simulink model "simulink_test"  (R2022b)
settings: Solver=VariableStepAuto  StartTime=0.0  StopTime=200000  RelTol=1e-3
undefined symbols (not defined in the file): m, n
settings Model: Creator=pedro  LastModifiedBy=pedro

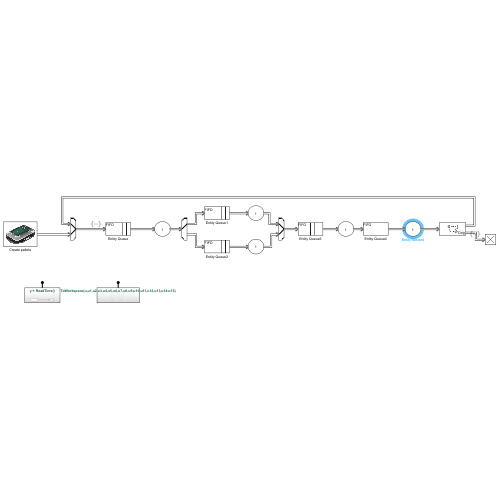
[thumbnail: Simulink's stored preview of the top-level diagram]
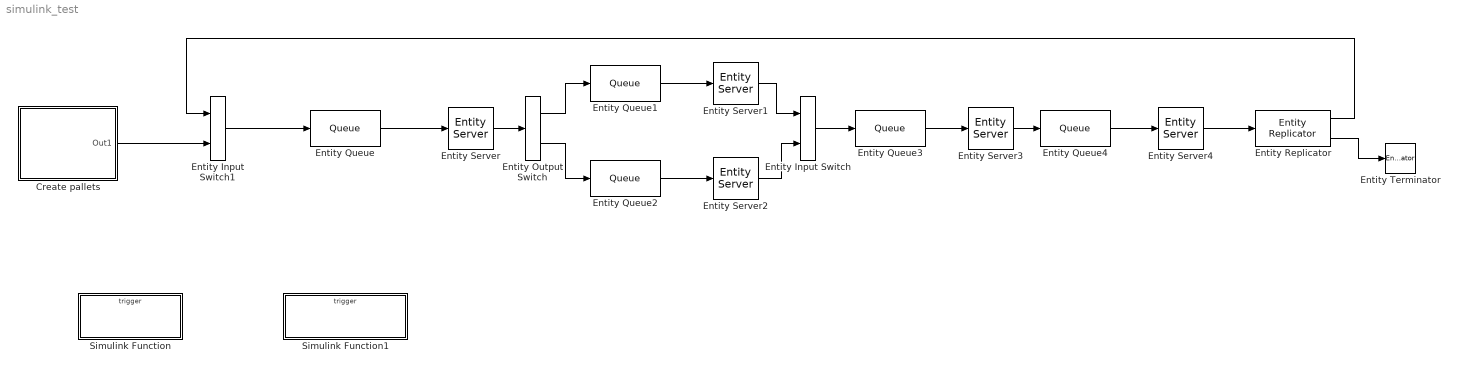
== system simulink_test ==
  Create pallets : Subsystem
      mask Display: image('$imagefile'); % Use "Edit Image" on toolstrip to change.
  Entity Input Switch : EntityInputSwitch  InputPortMessageModes=m,m  OutputPortMessageModes=m
  Entity Input Switch1 : EntityInputSwitch  InputPortMessageModes=m,m  OutputPortMessageModes=m
  Entity Output Switch : EntityOutputSwitch  InputPortMessageModes=m  OutputPortMessageModes=m,m  SwitchAttributeName=Attribute1
  Entity Queue : Queue  InputPortMessageModes=m  OutputPortMessageModes=m  Capacity=100  EntryAction=entity.Time_In_System = ReadTime();
  Entity Queue1 : Queue  InputPortMessageModes=m  OutputPortMessageModes=m  Capacity=3
  Entity Queue2 : Queue  InputPortMessageModes=m  OutputPortMessageModes=m  Capacity=7
  Entity Queue3 : Queue  InputPortMessageModes=m  OutputPortMessageModes=m  Capacity=20
  Entity Queue4 : Queue  InputPortMessageModes=m  OutputPortMessageModes=m  Capacity=10
  Entity Replicator : EntityReplicator  InputPortMessageModes=m  OutputPortMessageModes=m,m
  Entity Server : EntityServer  InputPortMessageModes=m  OutputPortMessageModes=m  Capacity=1  ServiceTimeValue=5000
  Entity Server1 : EntityServer  InputPortMessageModes=m  OutputPortMessageModes=m  Capacity=1  ServiceTimeValue=15000
  Entity Server2 : EntityServer  InputPortMessageModes=m  OutputPortMessageModes=m  Capacity=1  ServiceTimeValue=15000
  Entity Server3 : EntityServer  InputPortMessageModes=m  OutputPortMessageModes=m  Capacity=1  ServiceTimeValue=5000
  Entity Server4 : EntityServer  InputPortMessageModes=m  OutputPortMessageModes=m  Capacity=1  ServiceTimeValue=10000
  Entity Terminator : EntityTerminator  InputPortMessageModes=m  EntryAction=|
      | entity.Time_Out_System = ReadTime();
      | ToWorkspace(entity.Time_In_System,entity.Time_In_Cover, entity.Time_In_Drill, entity.Time_In_Robot, entity.Time_In_Camera, entity.Time_In_Back, entity.Time_In_Press, entity.Time_In_Manual, entity.Time_Out_System, entity.Time_Out_Cover, entity.Time_Out_Drill, entity.Time_Out_Robot, entity.Time_Out_Camera, entity.Time_Out_Back, entity.Time_Out_Press, entity.Time_Out_Manual)
  Simulink Function : Subsystem  TreatAsAtomicUnit=on
  Simulink Function1 : Subsystem  TreatAsAtomicUnit=on
  wires:
  Entity Queue/1 -> Entity Server/1
  Entity Server/1 -> Entity Output Switch/1
  Entity Output Switch/1 -> Entity Queue1/1
  Entity Output Switch/2 -> Entity Queue2/1
  Entity Queue1/1 -> Entity Server1/1
  Entity Queue2/1 -> Entity Server2/1
  Entity Server1/1 -> Entity Input Switch/1
  Entity Server2/1 -> Entity Input Switch/2
  Entity Input Switch/1 -> Entity Queue3/1
  Entity Queue3/1 -> Entity Server3/1
  Entity Server3/1 -> Entity Queue4/1
  Entity Queue4/1 -> Entity Server4/1
  Create pallets/1(Out1) -> Entity Input Switch1/2
  Entity Input Switch1/1 -> Entity Queue/1
  Entity Server4/1 -> Entity Replicator/1
  Entity Replicator/2 -> Entity Terminator/1
  Entity Replicator/1 -> Entity Input Switch1/1

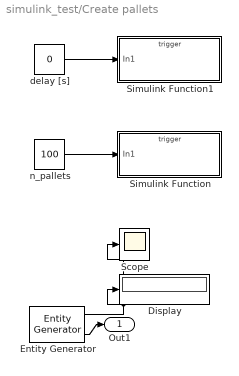
== system simulink_test/Create pallets ==
  Display : Display
  Entity Generator : EntityGenerator  OutputPortMessageModes=n,m  TimeSource=MATLAB action  IntergenerationTimeAction=|  GenerateEntityAtSimulationStart=off  GenerateAction=|  AttributeName=ID|Time_In_Cover|Time_Out_Cover|Time_In_Drill|Time_Out_Drill|Time_In_Robot|Time_Out_Robot|Time_In_Camera|Time_Out_Camera|Time_In_Back|Time_Out_Back|Time_In_Press|Time_Out_Press|Time_In_Manual|Time_Out_Manual|Time_Exit_Cover|Time_In_System|Time_Out_System|Queue1_capacity|Queue2_capacity|Queue3_capacity|Queue4_capacity|Queue5_capacity|Queue6_capacity|Queue1_time|Queue2_time|Queue3_time|Queue4_time|Queue5_time|Queue6_time|data30  AttributeInitialValue=1|0|0|0|0|0|0|0|0|0|0|0|0|0|0|0|0|0|1|1|1|1|1|1|1|1|1|1|1|1|1  NumberEntitiesDeparted=on  EntityType=Structured  EntityTypeName=Entity
      IntergenerationTimeAction=|
      | persistent count
      | if isempty(count)
      |     count = 1;
      | else
      |     count = count + 1;
      | end
      | dt = 0;
      | if count == 1
      |     dt = delay();
      | elseif count > n_pallets()
      |     dt = inf;
      | end
      GenerateAction=|
      | persistent count
      | if isempty(count)
      |     count = 1;
      | else
      |     count = count + 1;
      | end
      | entity.ID = count;
      settings: OutputPortMap=o0,o3
  Scope : Scope
  Simulink Function : Subsystem  TreatAsAtomicUnit=on
  Simulink Function1 : Subsystem  TreatAsAtomicUnit=on
  delay [s] : Constant  Value=0
  n_pallets : Constant  Value=100
  Out1 : Outport
  wires:
  Entity Generator/2 -> Out1/1
  Entity Generator/1 -> Display/1, Scope/1
  n_pallets/1 -> Simulink Function/1(In1)
  delay [s]/1 -> Simulink Function1/1(In1)

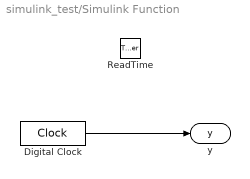
== system simulink_test/Simulink Function ==
  ReadTime : TriggerPort  TriggerType=function-call  IsSimulinkFunction=on  FunctionName=ReadTime  FunctionVisibility=scoped  VariantControl=(inherit)
  Digital Clock : DigitalClock  SampleTime=-1
  y : ArgOut  DisableCoverage=on  ArgumentName=y
  wires:
  Digital Clock/1 -> y/1

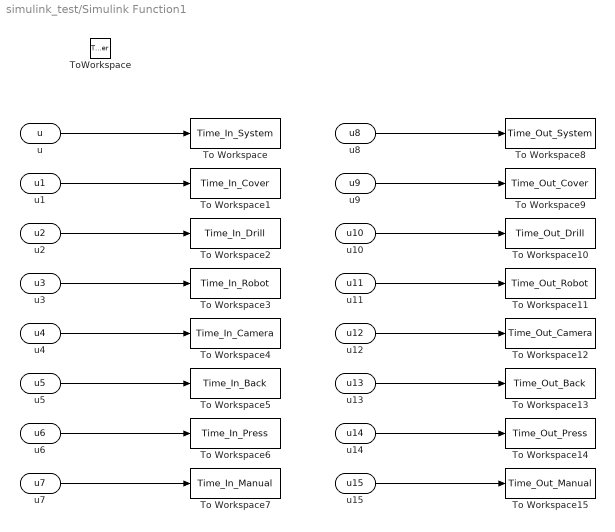
== system simulink_test/Simulink Function1 ==
  ToWorkspace : TriggerPort  TriggerType=function-call  IsSimulinkFunction=on  FunctionName=ToWorkspace  FunctionVisibility=scoped  VariantControl=(inherit)
  To Workspace : ToWorkspace  VariableName=Time_In_System  SampleTime=-1
      settings: Save2DSignal=2-D array (concatenate along first dimension)
  To Workspace1 : ToWorkspace  VariableName=Time_In_Cover  SampleTime=-1
      settings: Save2DSignal=2-D array (concatenate along first dimension)
  To Workspace10 : ToWorkspace  VariableName=Time_Out_Drill  SampleTime=-1
      settings: Save2DSignal=2-D array (concatenate along first dimension)
  To Workspace11 : ToWorkspace  VariableName=Time_Out_Robot  SampleTime=-1
      settings: Save2DSignal=2-D array (concatenate along first dimension)
  To Workspace12 : ToWorkspace  VariableName=Time_Out_Camera  SampleTime=-1
      settings: Save2DSignal=2-D array (concatenate along first dimension)
  To Workspace13 : ToWorkspace  VariableName=Time_Out_Back  SampleTime=-1
      settings: Save2DSignal=2-D array (concatenate along first dimension)
  To Workspace14 : ToWorkspace  VariableName=Time_Out_Press  SampleTime=-1
      settings: Save2DSignal=2-D array (concatenate along first dimension)
  To Workspace15 : ToWorkspace  VariableName=Time_Out_Manual  SampleTime=-1
      settings: Save2DSignal=2-D array (concatenate along first dimension)
  To Workspace2 : ToWorkspace  VariableName=Time_In_Drill  SampleTime=-1
      settings: Save2DSignal=2-D array (concatenate along first dimension)
  To Workspace3 : ToWorkspace  VariableName=Time_In_Robot  SampleTime=-1
      settings: Save2DSignal=2-D array (concatenate along first dimension)
  To Workspace4 : ToWorkspace  VariableName=Time_In_Camera  SampleTime=-1
      settings: Save2DSignal=2-D array (concatenate along first dimension)
  To Workspace5 : ToWorkspace  VariableName=Time_In_Back  SampleTime=-1
      settings: Save2DSignal=2-D array (concatenate along first dimension)
  To Workspace6 : ToWorkspace  VariableName=Time_In_Press  SampleTime=-1
      settings: Save2DSignal=2-D array (concatenate along first dimension)
  To Workspace7 : ToWorkspace  VariableName=Time_In_Manual  SampleTime=-1
      settings: Save2DSignal=2-D array (concatenate along first dimension)
  To Workspace8 : ToWorkspace  VariableName=Time_Out_System  SampleTime=-1
      settings: Save2DSignal=2-D array (concatenate along first dimension)
  To Workspace9 : ToWorkspace  VariableName=Time_Out_Cover  SampleTime=-1
      settings: Save2DSignal=2-D array (concatenate along first dimension)
  u : ArgIn  DisableCoverage=on  ArgumentName=u
  u1 : ArgIn  DisableCoverage=on  Port=2  ArgumentName=u1
  u2 : ArgIn  DisableCoverage=on  Port=3  ArgumentName=u2
  u3 : ArgIn  DisableCoverage=on  Port=4  ArgumentName=u3
  u4 : ArgIn  DisableCoverage=on  Port=5  ArgumentName=u4
  u5 : ArgIn  DisableCoverage=on  Port=6  ArgumentName=u5
  u6 : ArgIn  DisableCoverage=on  Port=7  ArgumentName=u6
  u7 : ArgIn  DisableCoverage=on  Port=8  ArgumentName=u7
  u8 : ArgIn  DisableCoverage=on  Port=9  ArgumentName=u8
  u9 : ArgIn  DisableCoverage=on  Port=10  ArgumentName=u9
  u10 : ArgIn  DisableCoverage=on  Port=11  ArgumentName=u10
  u11 : ArgIn  DisableCoverage=on  Port=12  ArgumentName=u11
  u12 : ArgIn  DisableCoverage=on  Port=13  ArgumentName=u12
  u13 : ArgIn  DisableCoverage=on  Port=14  ArgumentName=u13
  u14 : ArgIn  DisableCoverage=on  Port=15  ArgumentName=u14
  u15 : ArgIn  DisableCoverage=on  Port=16  ArgumentName=u15
  wires:
  u/1 -> To Workspace/1
  u1/1 -> To Workspace1/1
  u2/1 -> To Workspace2/1
  u3/1 -> To Workspace3/1
  u6/1 -> To Workspace6/1
  u5/1 -> To Workspace5/1
  u7/1 -> To Workspace7/1
  u4/1 -> To Workspace4/1
  u12/1 -> To Workspace12/1
  u15/1 -> To Workspace15/1
  u10/1 -> To Workspace10/1
  u13/1 -> To Workspace13/1
  u9/1 -> To Workspace9/1
  u14/1 -> To Workspace14/1
  u11/1 -> To Workspace11/1
  u8/1 -> To Workspace8/1

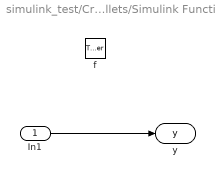
== system simulink_test/Create pallets/Simulink Function ==
  In1 : Inport
  f : TriggerPort  TriggerType=function-call  IsSimulinkFunction=on  FunctionName=n_pallets  FunctionVisibility=scoped  VariantControl=(inherit)
  y : ArgOut  DisableCoverage=on  ArgumentName=y
  wires:
  In1/1 -> y/1

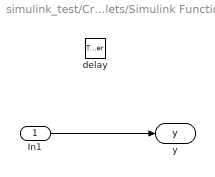
== system simulink_test/Create pallets/Simulink Function1 ==
  In1 : Inport
  delay : TriggerPort  TriggerType=function-call  IsSimulinkFunction=on  FunctionName=delay  FunctionVisibility=scoped  VariantControl=(inherit)
  y : ArgOut  DisableCoverage=on  ArgumentName=y
  wires:
  In1/1 -> y/1
